simulink model "jcc_ut"  (Simulink 8.1)
settings: Solver=FixedStepDiscrete  StartTime=0.0  StopTime=10  FixedStep=5E-3  RelTol=1e-3
PostLoadFcn:
  | , if any(exist('dsrtsu_mdlpostloadfcn', 'file') == [2, 3, 6]), try dsrtsu_mdlpostloadfcn('Execute', bdroot); catch fprintf('Error in PostLoadFcn (dsrtsu_mdlpostloadfcn) for model "%s":\n %s\n', bdroot, lasterr); end, end,
undefined symbols (not defined in the file or in its folder): VACC_ACCActing_flg, VACC_ACCOverride_flg, VACC_ACCRawTorqueReq_Nm, VACC_ACCSystemState_enum, VACC_DesiredDistance_m, VACC_StandstillClearance_m, VAEB_AEBActing_flg, VAEB_AEBSystemState_enum, VDHP_DisableACC_flg, VDHP_DisableADASFun_flg, VDINR_CurDriverTqReq_Nm, VDINR_DriverBrakPedalOn_flg, VDINR_HMICANValid_flg, VDINR_HWAccelPedalPosn_pct, VDINR_KeySwitchStatus_enum, VDINR_NowGearPosn_enum, VDINR_ParkBrakeBindSta_enum, VDINR_VehSpd_kph, VIFO_ACCCancelReq_flg, VIFO_ACCDist_flg, VIFO_ACCResSpdInc_flg, VIFO_ACCSetSpdDec_flg, VIFO_ACCTargetVehAssigned_flg, VIFO_ACCTargetVehRelSpeedX_mps, VIFO_ACCVehClearance_m, VIFO_DriverOvertakeReq_flg, VIFO_DriverSafetyStatusOk_flg, VIFO_DriverTurnSignalOn_flg, VIFO_VehicleStatusOk_flg, VPER_CameraStatus_enum, VPER_FusionStatus_enum, VPER_RadarStatus_enum
libraries: siltestlib x42, jcc x1
settings Model: DSRTSU_INTERNAL_RTI_VER=450  DSRTSU_INTERNAL_RTI_TYPE=rti1401  RTICANMMDATA=struct('GeneralSetupData',struct('modelroot','D:\ELN150201_TAIWAN\trunk\AdasDragon\software\sw_development\arch\app\jud','generalsettings',struct('filesettings',struct('destfolder',struct('Name','RTICANMM_FILES','Check',1),'buildfolder',struct('Name','.','Check',1),'AbsDestfolder',struct('Name','D:\ELN150201_TAIWAN\trunk\AdasDragon\software\sw_development\arch\app\jud\RTICANMM_FILES'),'AbsBuildfolder',struct('Name','D:\ELN150201_TAIWAN\trunk\AdasDragon\software\sw_development\arch\app\jud'))),'options',struct('addpaths',1,'rmpaths',1,'addtrcexclusion',logical(1),'cannavigator',struct('checkmonitoring',0),'show_usrtrc',0,'use_usrtrc',0),'advanced',struct('options',[1 1 1 1 1 1 1 1 1 1 1 1 1 1 1 1 1 1 1 1 1 1 1 1 1 1 1 1 1 1 1 1 1 1 1 1 1 1 1 1 1 1 1 1 1 1 1 1 1 1 1 1 1 1 1 1 1 1 1 1 1 1 1 1 1 1 1 1 1 1 1 1 1 1 1 1 1 1 1 1 1 1 1 1 1 1 1 1 1 1 1 1 1 1 1 1 1 1 1 1]),'MPSetup',{{}},'modelname','jcc_ut','block','jcc_ut'))  DSRTSU_INTERNAL_RTIFPGA=40  Creator=AT015411  LastModifiedBy=AT015555  BufferReuse=off
settings DataIOCC: SignalLoggingSaveFormat=Dataset
settings OptimizationCC: BlockReduction=off  OptimizeBlockIOStorage=off  BufferReuse=off  ExpressionFolding=off  ExpressionDepthLimit=128  LocalBlockOutputs=off
settings DebuggingCC: FcnCallInpInsideContextMsg=EnableAllAsError
settings HardwareCC: ProdIntDivRoundTo=Zero  ProdEndianess=BigEndian  ProdHWDeviceType=Generic->Custom  TargetIntDivRoundTo=Zero  TargetEndianess=BigEndian  TargetHWDeviceType=Generic->Custom
settings RTWCC: SystemTargetFile=rti1005.tlc  MakeCommand=make_rti  TemplateMakefile=rti1005.tmf  Description=dSPACE DS1005 Hardware Platform  ProcessScript=rti1005_make_rtw_hook
settings STFCustomTargetCC: CodeReplacementLibrary=ANSI_C  ParMdlRefBuildCompliant=on  GeneratePreprocessorConditionals=Disable all  MatFileLogging=on  SystemTargetFile=rti1005.tlc
settings GRTTargetCC: CompOptLevelCompliant=off  ConcurrentExecutionCompliant=off  ExtModeMexFile=noextcomm
settings CustomProperty: DataType=RTWOptions_EnumType_C__Program Files (x86)_dSPACE RCPHIL 2014-B_MATLAB_RTI_RTI1401_TLC_rti1005_1InitialSimState  Value=RUN
settings EnumStrPairs: String=RUN

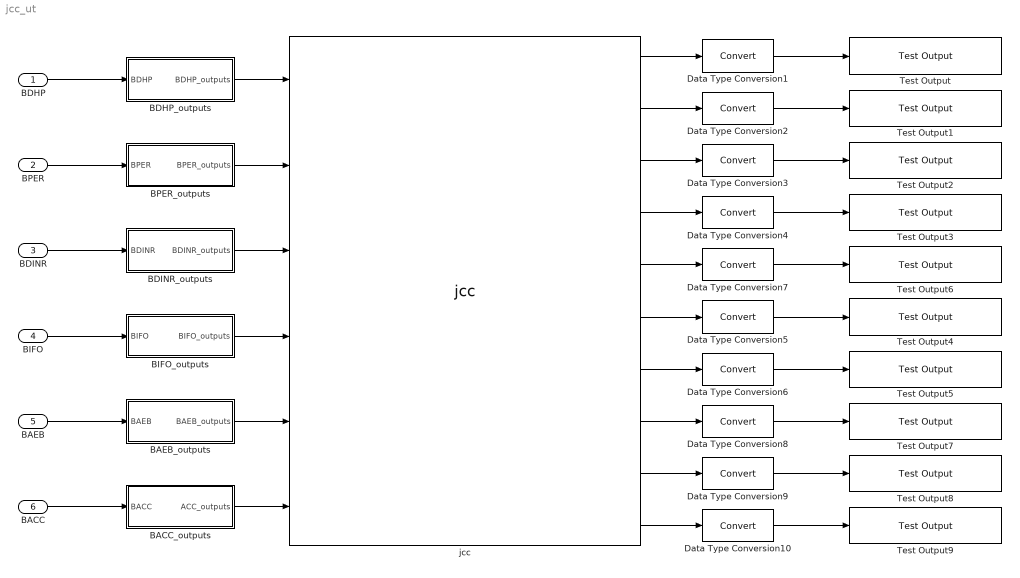
== system jcc_ut ==
  BDHP : Inport  OutDataTypeStr=Bus: BDHP_outputs
  BPER : Inport  Port=2  OutDataTypeStr=Bus: BPER_outputs
  BDINR : Inport  Port=3  OutDataTypeStr=Bus: BDINR_outputs
  BIFO : Inport  Port=4  OutDataTypeStr=Bus: BIFO_outputs
  BAEB : Inport  Port=5  OutDataTypeStr=Bus: BAEB_outputs
  BACC : Inport  Port=6  OutDataTypeStr=Bus: BACC_outputs
  BACC_outputs : Subsystem
  BAEB_outputs : Subsystem
  BDHP_outputs : Subsystem
  BDINR_outputs : Subsystem
  BIFO_outputs : Subsystem
  BPER_outputs : Subsystem
  Data Type Conversion{1..10} (10 alike) : DataTypeConversion
  Test Output : siltestlib/Test Output  varname=VJUD_ACCEnableReq_flg  sampletime=-1
  Test Output1 : siltestlib/Test Output  varname=VJUD_ACCActiveReq_flg  sampletime=-1
  Test Output2 : siltestlib/Test Output  varname=VJUD_ACCDeactivationReq_flg  sampletime=-1
  Test Output3 : siltestlib/Test Output  varname=VJUD_ACCStandstillReq_flg  sampletime=-1
  Test Output4 : siltestlib/Test Output  varname=VJUD_ACCOverrideReq_flg  sampletime=-1
  Test Output5 : siltestlib/Test Output  varname=VJUD_ACCSetSpeed_kph  sampletime=-1
  Test Output6 : siltestlib/Test Output  varname=VJUD_ACCRefollowReq_flg  sampletime=-1
  Test Output7 : siltestlib/Test Output  varname=VJUD_ACCSetTimeGap_s  sampletime=-1
  Test Output8 : siltestlib/Test Output  varname=VJUD_ACCHMISelTimeGap_s  sampletime=-1
  Test Output9 : siltestlib/Test Output  varname=VJUD_ACCSetSpeedSel_flg  sampletime=-1
  jcc : jcc/jcc
  wires:
  BDINR_outputs/1(BDINR_outputs) -> jcc/3
  BIFO_outputs/1(BIFO_outputs) -> jcc/4
  BPER_outputs/1(BPER_outputs) -> jcc/2
  BDINR/1 -> BDINR_outputs/1(BDINR)
  BPER/1 -> BPER_outputs/1(BPER)
  BIFO/1 -> BIFO_outputs/1(BIFO)
  BDHP_outputs/1(BDHP_outputs) -> jcc/1
  BDHP/1 -> BDHP_outputs/1(BDHP)
  BAEB_outputs/1(BAEB_outputs) -> jcc/5
  BAEB/1 -> BAEB_outputs/1(BAEB)
  Data Type Conversion1/1 -> Test Output/1
  Data Type Conversion2/1 -> Test Output1/1
  Data Type Conversion3/1 -> Test Output2/1
  Data Type Conversion4/1 -> Test Output3/1
  Data Type Conversion5/1 -> Test Output4/1
  Data Type Conversion6/1 -> Test Output5/1
  Data Type Conversion7/1 -> Test Output6/1
  BACC/1 -> BACC_outputs/1(BACC)
  BACC_outputs/1(ACC_outputs) -> jcc/6
  Data Type Conversion8/1 -> Test Output7/1
  Data Type Conversion9/1 -> Test Output8/1
  Data Type Conversion10/1 -> Test Output9/1
  jcc/1 -> Data Type Conversion1/1
  jcc/10 -> Data Type Conversion10/1
  jcc/2 -> Data Type Conversion2/1
  jcc/3 -> Data Type Conversion3/1
  jcc/4 -> Data Type Conversion4/1
  jcc/5 -> Data Type Conversion7/1
  jcc/6 -> Data Type Conversion5/1
  jcc/7 -> Data Type Conversion6/1
  jcc/8 -> Data Type Conversion8/1
  jcc/9 -> Data Type Conversion9/1

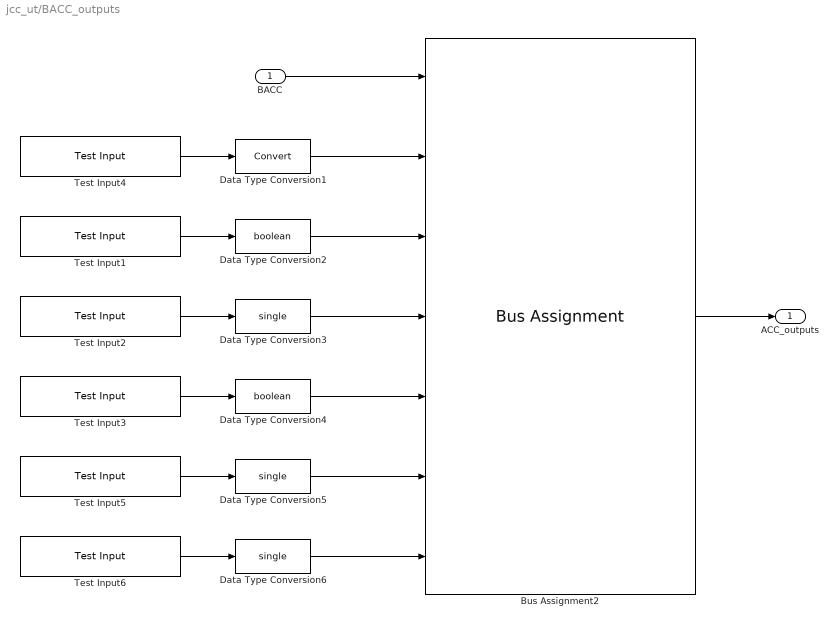
== system jcc_ut/BACC_outputs ==
  BACC : Inport  OutDataTypeStr=Bus: BACC_outputs
  Bus Assignment2 : BusAssignment  AssignedSignals=VACC_ACCSystemState_enum,VACC_ACCActing_flg,VACC_ACCRawTorqueReq_Nm,VACC_ACCOverride_flg,VACC_DesiredDistance_m,VACC_StandstillClearance_m
  Data Type Conversion1 : DataTypeConversion
  Data Type Conversion2 : DataTypeConversion  OutDataTypeStr=boolean
  Data Type Conversion3 : DataTypeConversion  OutDataTypeStr=single
  Data Type Conversion4 : DataTypeConversion  OutDataTypeStr=boolean
  Data Type Conversion5 : DataTypeConversion  OutDataTypeStr=single
  Data Type Conversion6 : DataTypeConversion  OutDataTypeStr=single
  Test Input1 : siltestlib/Test Input  varname=VACC_ACCActing_flg  sampletime=-1
  Test Input2 : siltestlib/Test Input  varname=VACC_ACCRawTorqueReq_Nm  sampletime=-1
  Test Input3 : siltestlib/Test Input  varname=VACC_ACCOverride_flg  sampletime=-1
  Test Input4 : siltestlib/Test Input  varname=VACC_ACCSystemState_enum  sampletime=-1
  Test Input5 : siltestlib/Test Input  varname=VACC_DesiredDistance_m  sampletime=-1
  Test Input6 : siltestlib/Test Input  varname=VACC_StandstillClearance_m  sampletime=-1
  ACC_outputs : Outport  OutDataTypeStr=Bus: BAEB_outputs
  wires:
  Test Input4/1 -> Data Type Conversion1/1
  Bus Assignment2/1 -> ACC_outputs/1
  BACC/1 -> Bus Assignment2/1
  Test Input1/1 -> Data Type Conversion2/1
  Test Input2/1 -> Data Type Conversion3/1
  Test Input3/1 -> Data Type Conversion4/1
  Test Input5/1 -> Data Type Conversion5/1
  Test Input6/1 -> Data Type Conversion6/1
  Data Type Conversion1/1 -> Bus Assignment2/2
  Data Type Conversion6/1 -> Bus Assignment2/7
  Data Type Conversion2/1 -> Bus Assignment2/3
  Data Type Conversion5/1 -> Bus Assignment2/6
  Data Type Conversion4/1 -> Bus Assignment2/5
  Data Type Conversion3/1 -> Bus Assignment2/4

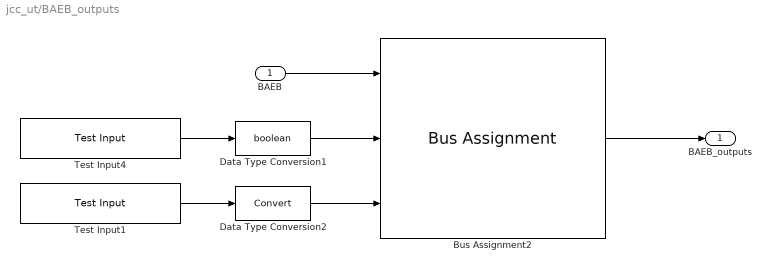
== system jcc_ut/BAEB_outputs ==
  BAEB : Inport  OutDataTypeStr=Bus: BAEB_outputs
  Bus Assignment2 : BusAssignment  AssignedSignals=VAEB_AEBActing_flg,VAEB_AEBSystemState_enum
  Data Type Conversion1 : DataTypeConversion  OutDataTypeStr=boolean
  Data Type Conversion2 : DataTypeConversion
  Test Input1 : siltestlib/Test Input  varname=VAEB_AEBSystemState_enum  sampletime=-1
  Test Input4 : siltestlib/Test Input  varname=VAEB_AEBActing_flg  sampletime=-1
  BAEB_outputs : Outport  OutDataTypeStr=Bus: BAEB_outputs
  wires:
  BAEB/1 -> Bus Assignment2/1
  Bus Assignment2/1 -> BAEB_outputs/1
  Test Input4/1 -> Data Type Conversion1/1
  Data Type Conversion1/1 -> Bus Assignment2/2
  Test Input1/1 -> Data Type Conversion2/1
  Data Type Conversion2/1 -> Bus Assignment2/3

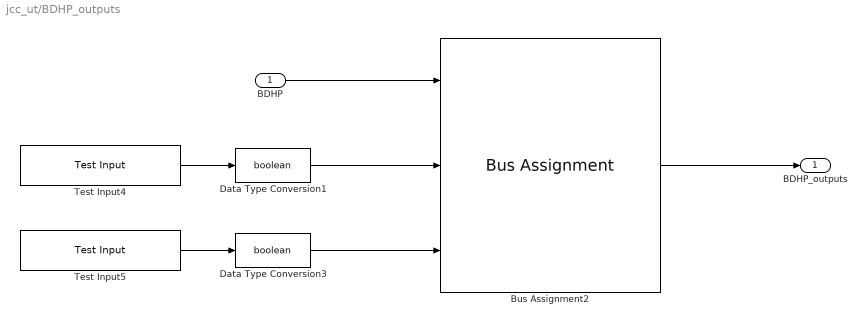
== system jcc_ut/BDHP_outputs ==
  BDHP : Inport  OutDataTypeStr=Bus: BDHP_outputs
  Bus Assignment2 : BusAssignment  AssignedSignals=VDHP_DisableADASFun_flg,VDHP_DisableACC_flg
  Data Type Conversion1 : DataTypeConversion  OutDataTypeStr=boolean
  Data Type Conversion3 : DataTypeConversion  OutDataTypeStr=boolean
  Test Input4 : siltestlib/Test Input  varname=VDHP_DisableADASFun_flg  sampletime=-1
  Test Input5 : siltestlib/Test Input  varname=VDHP_DisableACC_flg  sampletime=-1
  BDHP_outputs : Outport  OutDataTypeStr=Bus: BDHP_outputs
  wires:
  BDHP/1 -> Bus Assignment2/1
  Bus Assignment2/1 -> BDHP_outputs/1
  Test Input4/1 -> Data Type Conversion1/1
  Data Type Conversion1/1 -> Bus Assignment2/2
  Test Input5/1 -> Data Type Conversion3/1
  Data Type Conversion3/1 -> Bus Assignment2/3

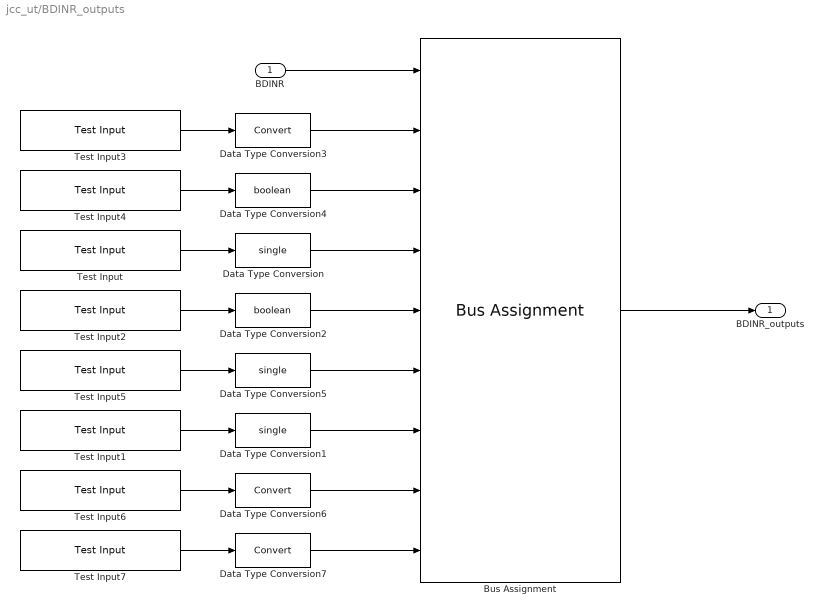
== system jcc_ut/BDINR_outputs ==
  BDINR : Inport  OutDataTypeStr=Bus: BDINR_outputs
  Bus Assignment : BusAssignment  AssignedSignals=VDINR_KeySwitchStatus_enum,VDINR_HMICANValid_flg,VDINR_VehSpd_kph,VDINR_DriverBrakPedalOn_flg,VDINR_HWAccelPedalPosn_pct,VDINR_CurDriverTqReq_Nm,VDINR_NowGearPosn_enum,VDINR_ParkBrakeBindSta_enum
  Data Type Conversion : DataTypeConversion  OutDataTypeStr=single
  Data Type Conversion1 : DataTypeConversion  OutDataTypeStr=single
  Data Type Conversion2 : DataTypeConversion  OutDataTypeStr=boolean
  Data Type Conversion3 : DataTypeConversion
  Data Type Conversion4 : DataTypeConversion  OutDataTypeStr=boolean
  Data Type Conversion5 : DataTypeConversion  OutDataTypeStr=single
  Data Type Conversion6 : DataTypeConversion
  Data Type Conversion7 : DataTypeConversion
  Test Input : siltestlib/Test Input  varname=VDINR_VehSpd_kph  sampletime=-1
  Test Input1 : siltestlib/Test Input  varname=VDINR_CurDriverTqReq_Nm  sampletime=-1
  Test Input2 : siltestlib/Test Input  varname=VDINR_DriverBrakPedalOn_flg  sampletime=-1
  Test Input3 : siltestlib/Test Input  varname=VDINR_KeySwitchStatus_enum  sampletime=-1
  Test Input4 : siltestlib/Test Input  varname=VDINR_HMICANValid_flg  sampletime=-1
  Test Input5 : siltestlib/Test Input  varname=VDINR_HWAccelPedalPosn_pct  sampletime=-1
  Test Input6 : siltestlib/Test Input  varname=VDINR_NowGearPosn_enum  sampletime=-1
  Test Input7 : siltestlib/Test Input  varname=VDINR_ParkBrakeBindSta_enum  sampletime=-1
  BDINR_outputs : Outport  OutDataTypeStr=Bus: BDINR_outputs
  wires:
  Bus Assignment/1 -> BDINR_outputs/1
  BDINR/1 -> Bus Assignment/1
  Test Input/1 -> Data Type Conversion/1
  Data Type Conversion/1 -> Bus Assignment/4
  Test Input1/1 -> Data Type Conversion1/1
  Data Type Conversion1/1 -> Bus Assignment/7
  Test Input2/1 -> Data Type Conversion2/1
  Data Type Conversion2/1 -> Bus Assignment/5
  Test Input3/1 -> Data Type Conversion3/1
  Data Type Conversion3/1 -> Bus Assignment/2
  Test Input4/1 -> Data Type Conversion4/1
  Data Type Conversion4/1 -> Bus Assignment/3
  Test Input5/1 -> Data Type Conversion5/1
  Data Type Conversion5/1 -> Bus Assignment/6
  Test Input6/1 -> Data Type Conversion6/1
  Data Type Conversion6/1 -> Bus Assignment/8
  Test Input7/1 -> Data Type Conversion7/1
  Data Type Conversion7/1 -> Bus Assignment/9

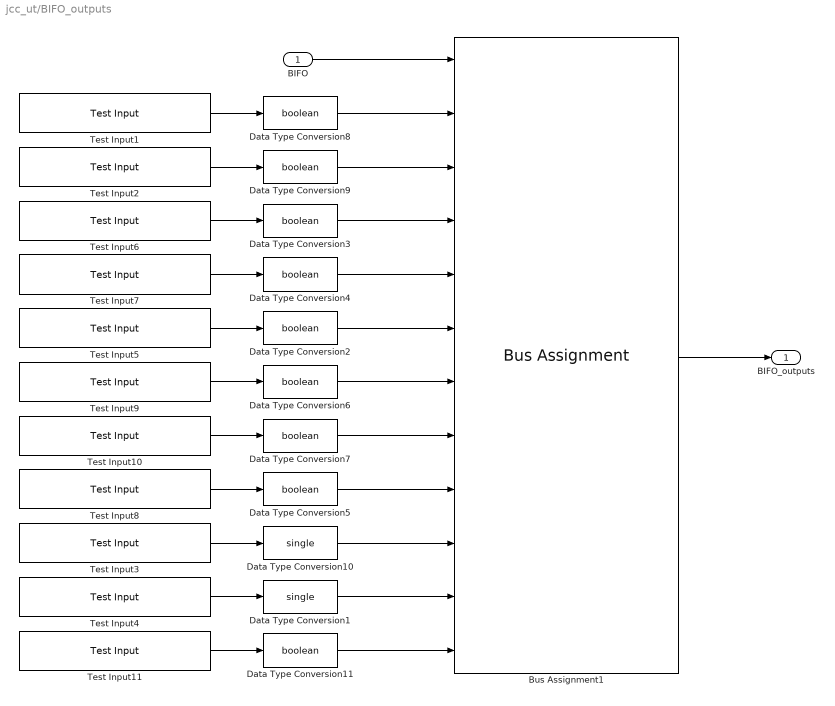
== system jcc_ut/BIFO_outputs ==
  BIFO : Inport  OutDataTypeStr=Bus: BIFO_outputs
  Bus Assignment1 : BusAssignment  AssignedSignals=VIFO_ACCSetSpdDec_flg,VIFO_ACCResSpdInc_flg,VIFO_ACCDist_flg,VIFO_ACCCancelReq_flg,VIFO_DriverOvertakeReq_flg,VIFO_VehicleStatusOk_flg,VIFO_DriverSafetyStatusOk_flg,VIFO_ACCTargetVehAssigned_flg,VIFO_ACCTargetVehRelSpeedX_mps,VIFO_ACCVehClearance_m,VIFO_DriverTurnSignalOn_flg
  Data Type Conversion1 : DataTypeConversion  OutDataTypeStr=single
  Data Type Conversion10 : DataTypeConversion  OutDataTypeStr=single
  Data Type Conversion{2..9,11} (9 alike) : DataTypeConversion  OutDataTypeStr=boolean
  Test Input1 : siltestlib/Test Input  varname=VIFO_ACCSetSpdDec_flg  sampletime=-1
  Test Input10 : siltestlib/Test Input  varname=VIFO_DriverSafetyStatusOk_flg  sampletime=-1
  Test Input11 : siltestlib/Test Input  varname=VIFO_DriverTurnSignalOn_flg  sampletime=-1
  Test Input2 : siltestlib/Test Input  varname=VIFO_ACCResSpdInc_flg  sampletime=-1
  Test Input3 : siltestlib/Test Input  varname=VIFO_ACCTargetVehRelSpeedX_mps  sampletime=-1
  Test Input4 : siltestlib/Test Input  varname=VIFO_ACCVehClearance_m  sampletime=-1
  Test Input5 : siltestlib/Test Input  varname=VIFO_DriverOvertakeReq_flg  sampletime=-1
  Test Input6 : siltestlib/Test Input  varname=VIFO_ACCDist_flg  sampletime=-1
  Test Input7 : siltestlib/Test Input  varname=VIFO_ACCCancelReq_flg  sampletime=-1
  Test Input8 : siltestlib/Test Input  varname=VIFO_ACCTargetVehAssigned_flg  sampletime=-1
  Test Input9 : siltestlib/Test Input  varname=VIFO_VehicleStatusOk_flg  sampletime=-1
  BIFO_outputs : Outport  OutDataTypeStr=Bus: BIFO_outputs
  wires:
  BIFO/1 -> Bus Assignment1/1
  Bus Assignment1/1 -> BIFO_outputs/1
  Test Input1/1 -> Data Type Conversion8/1
  Data Type Conversion8/1 -> Bus Assignment1/2
  Test Input2/1 -> Data Type Conversion9/1
  Data Type Conversion9/1 -> Bus Assignment1/3
  Test Input3/1 -> Data Type Conversion10/1
  Data Type Conversion3/1 -> Bus Assignment1/4
  Test Input4/1 -> Data Type Conversion1/1
  Data Type Conversion1/1 -> Bus Assignment1/11
  Data Type Conversion10/1 -> Bus Assignment1/10
  Test Input5/1 -> Data Type Conversion2/1
  Data Type Conversion2/1 -> Bus Assignment1/6
  Test Input6/1 -> Data Type Conversion3/1
  Data Type Conversion4/1 -> Bus Assignment1/5
  Test Input7/1 -> Data Type Conversion4/1
  Data Type Conversion5/1 -> Bus Assignment1/9
  Test Input8/1 -> Data Type Conversion5/1
  Data Type Conversion6/1 -> Bus Assignment1/7
  Test Input9/1 -> Data Type Conversion6/1
  Data Type Conversion7/1 -> Bus Assignment1/8
  Test Input10/1 -> Data Type Conversion7/1
  Test Input11/1 -> Data Type Conversion11/1
  Data Type Conversion11/1 -> Bus Assignment1/12

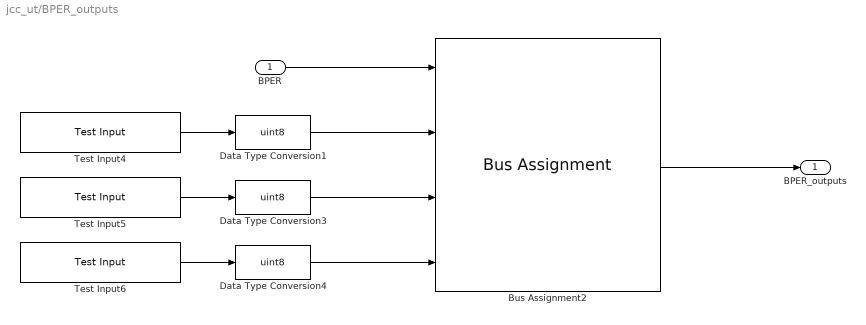
== system jcc_ut/BPER_outputs ==
  BPER : Inport  OutDataTypeStr=Bus: BPER_outputs
  Bus Assignment2 : BusAssignment  AssignedSignals=VPER_CameraStatus_enum,VPER_RadarStatus_enum,VPER_FusionStatus_enum
  Data Type Conversion1 : DataTypeConversion  OutDataTypeStr=uint8
  Data Type Conversion3 : DataTypeConversion  OutDataTypeStr=uint8
  Data Type Conversion4 : DataTypeConversion  OutDataTypeStr=uint8
  Test Input4 : siltestlib/Test Input  varname=VPER_CameraStatus_enum  sampletime=-1
  Test Input5 : siltestlib/Test Input  varname=VPER_RadarStatus_enum  sampletime=-1
  Test Input6 : siltestlib/Test Input  varname=VPER_FusionStatus_enum  sampletime=-1
  BPER_outputs : Outport  OutDataTypeStr=Bus: BPER_outputs
  wires:
  BPER/1 -> Bus Assignment2/1
  Bus Assignment2/1 -> BPER_outputs/1
  Test Input4/1 -> Data Type Conversion1/1
  Data Type Conversion1/1 -> Bus Assignment2/2
  Test Input5/1 -> Data Type Conversion3/1
  Data Type Conversion3/1 -> Bus Assignment2/3
  Test Input6/1 -> Data Type Conversion4/1
  Data Type Conversion4/1 -> Bus Assignment2/4
